simulink model "compensator"  (R2025b)
settings: Solver=ode14x  StartTime=0.0  StopTime=20  FixedStep=Ts_local  RelTol=1e-3
model workspace (MAT data in the model file):
  delta = 0.005
  u_d = 0.093
  v_a = -0.1537
  v_b = -0.1535
undefined symbols (not defined in the file or in its folder): lut_speed, lut_voltage, u_lb, u_ub
libraries: simulink x3
settings Model: DataDictionary=ctrlSys.sldd  Creator=mercer  LastModifiedBy=mercer

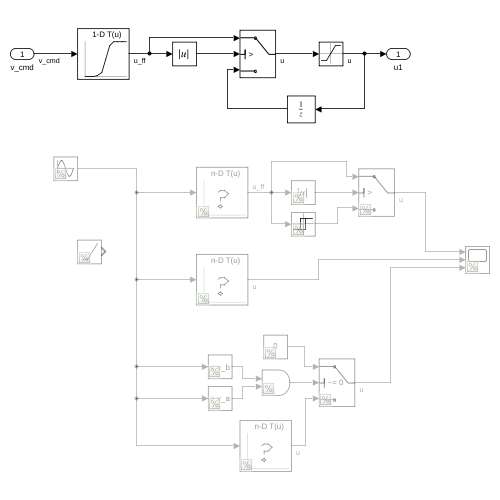
[thumbnail: Simulink's stored preview of the top-level diagram]
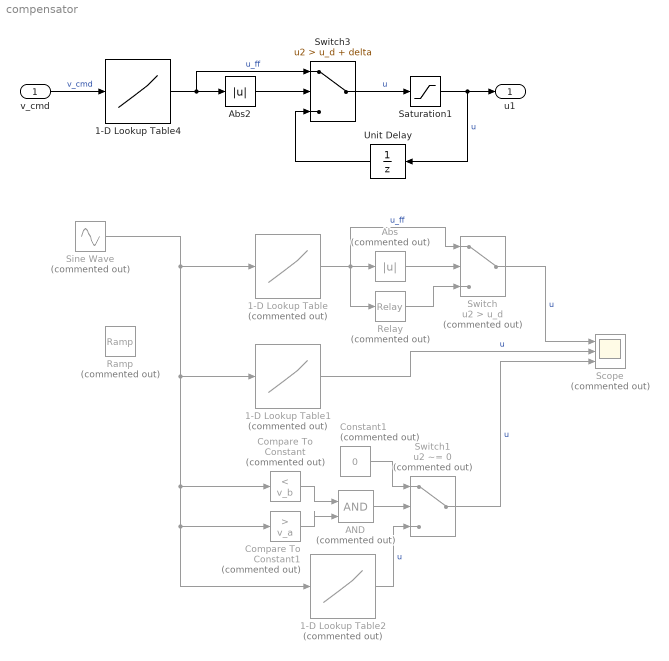
== system compensator ==
  v_cmd : Inport  PortDimensions=3
  1-D Lookup Table : Lookup_n-D  Commented=on  NumberOfTableDimensions=1  BreakpointsForDimension1=lut_speed  Table=lut_voltage  ExtrapMethod=Clip  InternalRulePriority=Speed  RndMeth=Simplest
  1-D Lookup Table1 : Lookup_n-D  Commented=on  NumberOfTableDimensions=1  BreakpointsForDimension1=lut_speed  Table=lut_voltage  ExtrapMethod=Clip  InternalRulePriority=Speed  RndMeth=Simplest
  1-D Lookup Table2 : Lookup_n-D  Commented=on  NumberOfTableDimensions=1  BreakpointsForDimension1=lut_speed  Table=lut_voltage  ExtrapMethod=Clip  InternalRulePriority=Speed  RndMeth=Simplest
  1-D Lookup Table4 : Lookup_n-D  NumberOfTableDimensions=1  BreakpointsForDimension1=lut_speed  Table=lut_voltage  ExtrapMethod=Clip  InternalRulePriority=Speed  RndMeth=Simplest
  AND : Logic  Commented=on  IconShape=distinctive  AllPortsSameDT=off  OutDataTypeStr=boolean
  Abs : Abs  Commented=on  SaturateOnIntegerOverflow=off
  Abs2 : Abs  SaturateOnIntegerOverflow=off
  Compare To Constant : simulink/Logic and Bit Operations/Compare To Constant  Commented=on  relop=<  const=v_b  OutDataTypeStr=boolean
  Compare To Constant1 : simulink/Logic and Bit Operations/Compare To Constant  Commented=on  relop=>  const=v_a  OutDataTypeStr=boolean
  Constant1 : Constant  Commented=on  Value=0
  Ramp : simulink/Sources/Ramp  Commented=on  slope=(0.2 - (-0.4)) / 100  start=0  InitialOutput=-0.4
  Relay : Relay  Commented=on  OnSwitchValue=u_d  OffSwitchValue=-u_d  OnOutputValue=u_d  OffOutputValue=-u_d
  Saturation1 : Saturate  UpperLimit=u_ub  LowerLimit=u_lb
  Scope : Scope  Commented=on  NumInputPorts=3
      settings: ActiveDisplayYMinimum=-0.1228099391587118  ActiveDisplayYMaximum=0.12031101740767525
  Sine Wave : Sin  Commented=on  Amplitude=0.001  Bias=-0.1536  SampleTime=0
  Switch : Switch  Commented=on  Criteria=u2 > Threshold  Threshold=u_d  SaturateOnIntegerOverflow=off  InputSameDT=off
  Switch1 : Switch  Commented=on  Criteria=u2 ~= 0  Threshold=u_d  SaturateOnIntegerOverflow=off  InputSameDT=off
  Switch3 : Switch  Criteria=u2 > Threshold  Threshold=u_d + delta  SaturateOnIntegerOverflow=off  InputSameDT=off
  Unit Delay : UnitDelay  SampleTime=-1  HasFrameUpgradeWarning=on
  u1 : Outport
  wires:
  1-D Lookup Table/1 -> Relay/1, Switch/1, Abs/1  "u_ff"
  Compare To Constant/1 -> AND/1
  Compare To Constant1/1 -> AND/2
  AND/1 -> Switch1/2
  Switch/1 -> Scope/1  "u"
  1-D Lookup Table1/1 -> Scope/2  "u"
  Abs/1 -> Switch/2
  Constant1/1 -> Switch1/1
  1-D Lookup Table2/1 -> Switch1/3  "u"
  Switch1/1 -> Scope/3  "u"
  Relay/1 -> Switch/3
  Sine Wave/1 -> 1-D Lookup Table2/1, Compare To Constant1/1, Compare To Constant/1, 1-D Lookup Table1/1, 1-D Lookup Table/1
  1-D Lookup Table4/1 -> Switch3/1, Abs2/1  "u_ff"
  Abs2/1 -> Switch3/2
  Switch3/1 -> Saturation1/1  "u"
  Saturation1/1 -> Unit Delay/1, u1/1  "u"
  Unit Delay/1 -> Switch3/3
  v_cmd/1 -> 1-D Lookup Table4/1  "v_cmd"
